simulink model "Selector_verif"  (Simulink 7.2)
settings: Solver=ode45  StartTime=0.0  StopTime=10.0  RelTol=1e-3
settings Model: Creator=Romain  LastModifiedBy=Romain
settings OptimizationCC: ExpressionDepthLimit=128
settings DebuggingCC: SolverPrmCheckMsg=none  FcnCallInpInsideContextMsg=Enable All  StateNameClashWarn=none  StrictBusMsg=ErrorLevel1
settings CodeAppCC: CustomSymbolStrType=$N$R$M_T
settings GRTTargetCC: TargetFunctionLibrary=C89/C90 (ANSI)

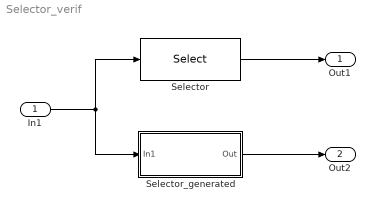
== system Selector_verif ==
  In1 : Inport  OutDataTypeStr=double  DataType=double
  Selector : Selector  InputPortWidth=3  Indices=[1 3]
  Selector_generated : Subsystem  TreatAsAtomicUnit=on
  Out1 : Outport
  Out2 : Outport  Port=2
  wires:
  In1/1 -> Selector_generated/1(In1), Selector/1
  Selector/1 -> Out1/1
  Selector_generated/1(Out) -> Out2/1

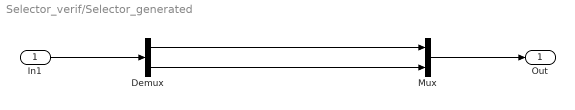
== system Selector_verif/Selector_generated ==
  In1 : Inport
  Demux : Demux  Outputs=3
  Mux : Mux  Inputs=2
  Out : Outport  RequirementInfo={} %GIDa_dcf46fcd_4a6e_48ca_9d55_6b4bd77be974
  wires:
  In1/1 -> Demux/1
  Mux/1 -> Out/1
  Demux/1 -> Mux/1
  Demux/3 -> Mux/2
